simulink model "SelfBalancingRobotTransferFunction"  (R2022b)
settings: Solver=FixedStepAuto  StartTime=0.0  StopTime=20  FixedStep=0.01  RelTol=1e-3
settings Model: Creator=Admins  LastModifiedBy=Admins
settings DataIOCC: ReturnWorkspaceOutputs=off

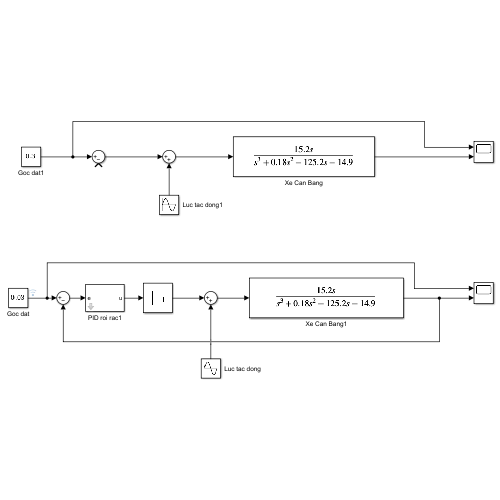
[thumbnail: Simulink's stored preview of the top-level diagram]
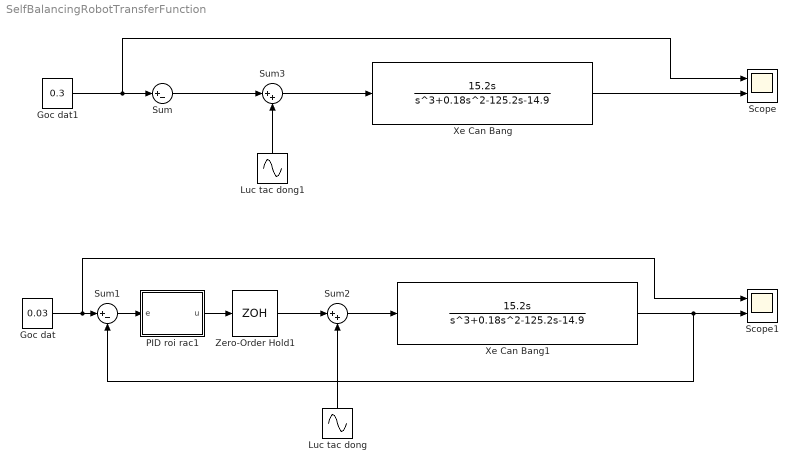
== system SelfBalancingRobotTransferFunction ==
  Goc dat : Constant  Value=0.03  SampleTime=0.01
  Goc dat1 : Constant  Value=0.3  SampleTime=0.01
  Luc tac dong : Sin  SampleTime=0
  Luc tac dong1 : Sin  SampleTime=0
  PID roi rac1 : Subsystem  mask{Kp=50, Ki=100, Kd=2, T=0.01}
  Scope : Scope  NumInputPorts=2
  Scope1 : Scope  NumInputPorts=2
  Sum : Sum  Inputs=|+-
  Sum1 : Sum  Inputs=|+-
  Sum2 : Sum  Inputs=|++
  Sum3 : Sum  Inputs=|++
  Xe Can Bang : TransferFcn  Numerator=[15.2 0]  Denominator=[1 0.18 -125.2 -14.9]
  Xe Can Bang1 : TransferFcn  Numerator=[15.2 0]  Denominator=[1 0.18 -125.2 -14.9]
  Zero-Order Hold1 : ZeroOrderHold  SampleTime=0.01
  wires:
  Xe Can Bang/1 -> Scope/2
  Goc dat1/1 -> Scope/1, Sum/1
  PID roi rac1/1(u) -> Zero-Order Hold1/1
  Sum1/1 -> PID roi rac1/1(e)
  Zero-Order Hold1/1 -> Sum2/1
  Xe Can Bang1/1 -> Sum1/2, Scope1/2
  Goc dat/1 -> Scope1/1, Sum1/1
  Sum2/1 -> Xe Can Bang1/1
  Luc tac dong/1 -> Sum2/2
  Luc tac dong1/1 -> Sum3/2
  Sum3/1 -> Xe Can Bang/1
  Sum/1 -> Sum3/1

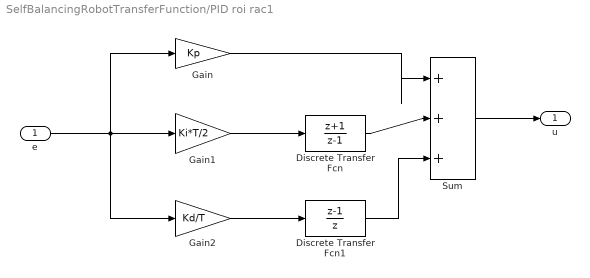
== system SelfBalancingRobotTransferFunction/PID roi rac1 ==
  e : Inport
  Discrete Transfer Fcn : DiscreteTransferFcn  Numerator=[1 1]  Denominator=[1 -1]
  Discrete Transfer Fcn1 : DiscreteTransferFcn  Numerator=[1 -1]  Denominator=[1 0]
  Gain : Gain  Gain=Kp
  Gain1 : Gain  Gain=Ki*T/2
  Gain2 : Gain  Gain=Kd/T
  Sum : Sum  Inputs=|+++
  u : Outport
  wires:
  e/1 -> Gain2/1, Gain1/1, Gain/1
  Gain1/1 -> Discrete Transfer Fcn/1
  Gain2/1 -> Discrete Transfer Fcn1/1
  Discrete Transfer Fcn1/1 -> Sum/3
  Discrete Transfer Fcn/1 -> Sum/2
  Gain/1 -> Sum/1
  Sum/1 -> u/1
